simulink model "ArchModel"  (R2022a)
settings: Solver=VariableStepAuto  StartTime=0.0  StopTime=10.0  RelTol=1e-3
undefined symbols (not defined in the file or in its folder): Neg, Pos
undefined symbols (not defined in the file): DCL, EIS
settings Model: DataDictionary=DesignDictionary.sldd  Creator=mateu  LastModifiedBy=mateu

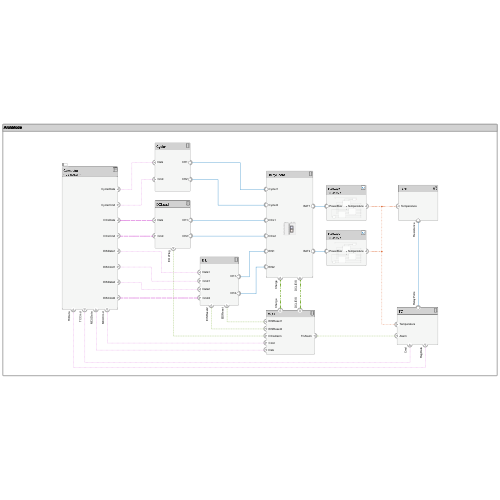
[thumbnail: Simulink's stored preview of the top-level diagram]
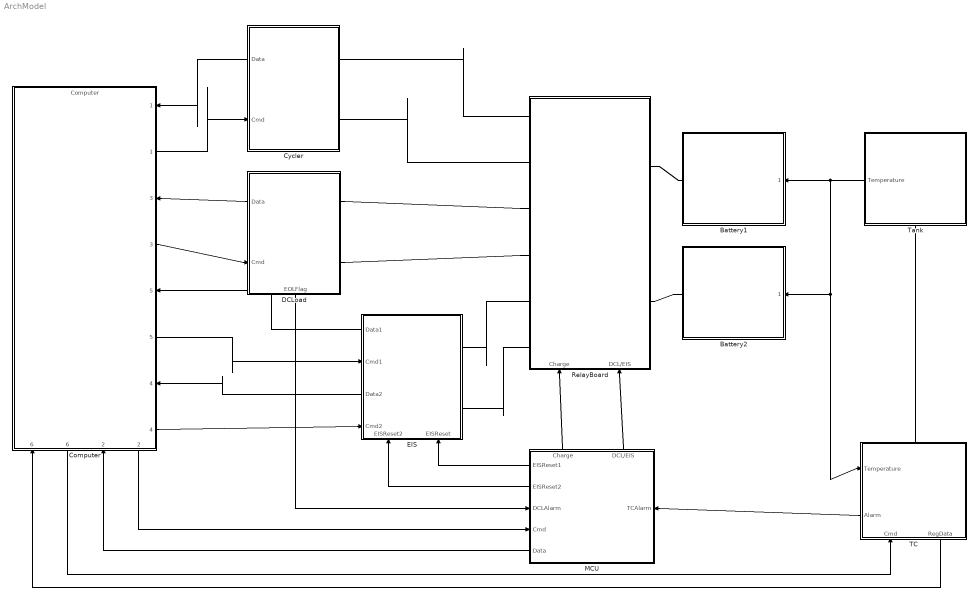
== system ArchModel ==
  Battery1 : Subsystem  ReferencedSubsystem=Battery
      settings: PortSchema="{\"entries\":[{\"content\":{\"headerSize\":26,\"margin\":15,\"minimumSpacing\":25,\"sides\":[{\"content\":{\"connectorIds\":[\"LConn1\"]},\"type\":\"ConnectorPlacement.EquallySpacedRectSide\",\"uuid\":\"7293e18d-b59a-4d1c-a013-b44ef7d38755\"},{\"content\":{\"connectorIds\":[\"In1\"],\"side\":\"RIGHT\"},\"type\":\"ConnectorPlacement.EquallySpacedRectSide\",\"uuid\":\"db41c958-7f9e-4f99-af5d-e3693d871bc2\"},{\"content\":{\"connectorIds\":[],\"side\":\"TOP\"},\"type\":\"ConnectorPlacement.EquallySpacedRectSide\",\"uuid\":\"914cc5b9-3cb5-4f98-b1a2-289c6929f7e4\"}]},\"type\":\"ConnectorPlacement.EquallySpacedConnector\",\"uuid\":\"372b3388-b57b-4345-a443-2207ebd52313\"}],\"packageUris\":[\"http://schema.mathworks.com/mf0/Connector/R2020b\"],\"version\":\"1.0\"}"
  Battery2 : Subsystem  ReferencedSubsystem=Battery
      settings: PortSchema="{\"entries\":[{\"content\":{\"headerSize\":26,\"margin\":15,\"minimumSpacing\":25,\"sides\":[{\"content\":{\"connectorIds\":[\"LConn1\"]},\"type\":\"ConnectorPlacement.EquallySpacedRectSide\",\"uuid\":\"7293e18d-b59a-4d1c-a013-b44ef7d38755\"},{\"content\":{\"connectorIds\":[\"In1\"],\"side\":\"RIGHT\"},\"type\":\"ConnectorPlacement.EquallySpacedRectSide\",\"uuid\":\"db41c958-7f9e-4f99-af5d-e3693d871bc2\"},{\"content\":{\"connectorIds\":[],\"side\":\"TOP\"},\"type\":\"ConnectorPlacement.EquallySpacedRectSide\",\"uuid\":\"914cc5b9-3cb5-4f98-b1a2-289c6929f7e4\"}]},\"type\":\"ConnectorPlacement.EquallySpacedConnector\",\"uuid\":\"372b3388-b57b-4345-a443-2207ebd52313\"}],\"packageUris\":[\"http://schema.mathworks.com/mf0/Connector/R2020b\"],\"version\":\"1.0\"}"
  Computer : ModelReference  ModelNameDialog=Computer  SimulationMode=Normal  ScheduleRates=on  ScheduleRatesWith=Schedule Editor  ModelReferenceVersion=1.3
      settings: PortSchema="{\"entries\":[{\"content\":{\"headerSize\":38,\"margin\":15,\"minimumSpacing\":25,\"sides\":[{\"content\":{\"connectorIds\":[]},\"type\":\"ConnectorPlacement.EquallySpacedRectSide\",\"uuid\":\"7293e18d-b59a-4d1c-a013-b44ef7d38755\"},{\"content\":{\"connectorIds\":[\"In1\",\"Out1\",\"In3\",\"Out3\",\"In5\",\"Out5\",\"In4\",\"Out4\"],\"side\":\"RIGHT\"},\"type\":\"ConnectorPlacement.EquallySpacedRectSide\",\"uuid\":\"db41c958-7f9e-4f99-af5d-e3693d871bc2\"},{\"content\":{\"connectorIds\":[],\"side\":\"TOP\"},\"type\":\"ConnectorPlacement.EquallySpacedRectSide\",\"uuid\":\"914cc5b9-3cb5-4f98-b1a2-289c6929f7e4\"},{\"content\":{\"connectorIds\":[\"In6\",\"Out6\",\"In2\",\"Out2\"],\"side\":\"BOTTOM\"},\"type\":\"ConnectorPlacement.EquallySpacedRectSide\",\"uuid\":\"ba0d90bc-7736-41e6-82f3-c99b67a5d224\"}]},\"type\":\"ConnectorPlacement.EquallySpacedConnector\",\"uuid\":\"372b3388-b57b-4345-a443-2207ebd52313\"}],\"packageUris\":[\"http://schema.mathworks.com/mf0/Connector/R2020b\"],\"version\":\"1.0\"}"
  Cycler : Subsystem
      settings: PortSchema="{\"entries\":[{\"content\":{\"headerSize\":26,\"margin\":15,\"minimumSpacing\":25,\"sides\":[{\"content\":{\"connectorIds\":[\"Out1\",\"In1\"]},\"type\":\"ConnectorPlacement.EquallySpacedRectSide\",\"uuid\":\"7293e18d-b59a-4d1c-a013-b44ef7d38755\"},{\"content\":{\"connectorIds\":[\"RConn1\",\"RConn2\"],\"side\":\"RIGHT\"},\"type\":\"ConnectorPlacement.EquallySpacedRectSide\",\"uuid\":\"db41c958-7f9e-4f99-af5d-e3693d871bc2\"},{\"content\":{\"connectorIds\":[],\"side\":\"TOP\"},\"type\":\"ConnectorPlacement.EquallySpacedRectSide\",\"uuid\":\"914cc5b9-3cb5-4f98-b1a2-289c6929f7e4\"}]},\"type\":\"ConnectorPlacement.EquallySpacedConnector\",\"uuid\":\"372b3388-b57b-4345-a443-2207ebd52313\"}],\"packageUris\":[\"http://schema.mathworks.com/mf0/Connector/R2020b\"],\"version\":\"1.0\"}"
  DCLoad : Subsystem
      settings: PortSchema="{\"entries\":[{\"content\":{\"headerSize\":26,\"margin\":15,\"minimumSpacing\":25,\"sides\":[{\"content\":{\"connectorIds\":[\"Out2\",\"In1\"]},\"type\":\"ConnectorPlacement.EquallySpacedRectSide\",\"uuid\":\"7293e18d-b59a-4d1c-a013-b44ef7d38755\"},{\"content\":{\"connectorIds\":[\"RConn1\",\"RConn2\"],\"side\":\"RIGHT\"},\"type\":\"ConnectorPlacement.EquallySpacedRectSide\",\"uuid\":\"db41c958-7f9e-4f99-af5d-e3693d871bc2\"},{\"content\":{\"connectorIds\":[],\"side\":\"TOP\"},\"type\":\"ConnectorPlacement.EquallySpacedRectSide\",\"uuid\":\"914cc5b9-3cb5-4f98-b1a2-289c6929f7e4\"},{\"content\":{\"connectorIds\":[\"Out1\"],\"side\":\"BOTTOM\"},\"type\":\"ConnectorPlacement.EquallySpacedRectSide\",\"uuid\":\"1b886045-7e55-48a4-a5ee-d0c1d4827f52\"}]},\"type\":\"ConnectorPlacement.EquallySpacedConnector\",\"uuid\":\"372b3388-b57b-4345-a443-2207ebd52313\"}],\"packageUris\":[\"http://schema.mathworks.com/mf0/Connector/R2020b\"],\"version\":\"1.0\"}"
  EIS : Subsystem
      settings: PortSchema="{\"entries\":[{\"content\":{\"headerSize\":26,\"margin\":15,\"minimumSpacing\":25,\"sides\":[{\"content\":{\"connectorIds\":[\"Out1\",\"In4\",\"Out2\",\"In3\"]},\"type\":\"ConnectorPlacement.EquallySpacedRectSide\",\"uuid\":\"7293e18d-b59a-4d1c-a013-b44ef7d38755\"},{\"content\":{\"connectorIds\":[\"RConn1\",\"RConn2\"],\"side\":\"RIGHT\"},\"type\":\"ConnectorPlacement.EquallySpacedRectSide\",\"uuid\":\"db41c958-7f9e-4f99-af5d-e3693d871bc2\"},{\"content\":{\"connectorIds\":[],\"side\":\"TOP\"},\"type\":\"ConnectorPlacement.EquallySpacedRectSide\",\"uuid\":\"914cc5b9-3cb5-4f98-b1a2-289c6929f7e4\"},{\"content\":{\"connectorIds\":[\"In1\",\"In2\"],\"side\":\"BOTTOM\"},\"type\":\"ConnectorPlacement.EquallySpacedRectSide\",\"uuid\":\"72880b12-21e3-4cc6-8f88-1609d84de5b0\"}]},\"type\":\"ConnectorPlacement.EquallySpacedConnector\",\"uuid\":\"372b3388-b57b-4345-a443-2207ebd52313\"}],\"packageUris\":[\"http://schema.mathworks.com/mf0/Connector/R2020b\"],\"version\":\"1.0\"}"
  MCU : Subsystem
      settings: PortSchema="{\"entries\":[{\"content\":{\"headerSize\":26,\"margin\":15,\"minimumSpacing\":25,\"sides\":[{\"content\":{\"connectorIds\":[\"Out1\",\"Out2\",\"In1\",\"In2\",\"Out3\"]},\"type\":\"ConnectorPlacement.EquallySpacedRectSide\",\"uuid\":\"7293e18d-b59a-4d1c-a013-b44ef7d38755\"},{\"content\":{\"connectorIds\":[\"In3\"],\"side\":\"RIGHT\"},\"type\":\"ConnectorPlacement.EquallySpacedRectSide\",\"uuid\":\"db41c958-7f9e-4f99-af5d-e3693d871bc2\"},{\"content\":{\"connectorIds\":[\"Out4\",\"Out5\"],\"side\":\"TOP\"},\"type\":\"ConnectorPlacement.EquallySpacedRectSide\",\"uuid\":\"914cc5b9-3cb5-4f98-b1a2-289c6929f7e4\"},{\"content\":{\"connectorIds\":[],\"side\":\"BOTTOM\"},\"type\":\"ConnectorPlacement.EquallySpacedRectSide\",\"uuid\":\"f4beb314-4f1a-4ac8-9406-4b22f31c5233\"}]},\"type\":\"ConnectorPlacement.EquallySpacedConnector\",\"uuid\":\"372b3388-b57b-4345-a443-2207ebd52313\"}],\"packageUris\":[\"http://schema.mathworks.com/mf0/Connector/R2020b\"],\"version\":\"1.0\"}"
  RelayBoard : Subsystem
      settings: PortSchema="{\"entries\":[{\"content\":{\"headerSize\":26,\"margin\":15,\"minimumSpacing\":25,\"sides\":[{\"content\":{\"connectorIds\":[\"LConn1\",\"LConn2\",\"LConn3\",\"LConn4\",\"LConn5\",\"LConn6\"]},\"type\":\"ConnectorPlacement.EquallySpacedRectSide\",\"uuid\":\"7293e18d-b59a-4d1c-a013-b44ef7d38755\"},{\"content\":{\"connectorIds\":[\"RConn1\",\"RConn2\"],\"side\":\"RIGHT\"},\"type\":\"ConnectorPlacement.EquallySpacedRectSide\",\"uuid\":\"db41c958-7f9e-4f99-af5d-e3693d871bc2\"},{\"content\":{\"connectorIds\":[],\"side\":\"TOP\"},\"type\":\"ConnectorPlacement.EquallySpacedRectSide\",\"uuid\":\"914cc5b9-3cb5-4f98-b1a2-289c6929f7e4\"},{\"content\":{\"connectorIds\":[\"In1\",\"In2\"],\"side\":\"BOTTOM\"},\"type\":\"ConnectorPlacement.EquallySpacedRectSide\",\"uuid\":\"a2b6a4b5-2cdb-4351-85fd-bf0b4fbbff2a\"}]},\"type\":\"ConnectorPlacement.EquallySpacedConnector\",\"uuid\":\"372b3388-b57b-4345-a443-2207ebd52313\"}],\"packageUris\":[\"http://schema.mathworks.com/mf0/Connector/R2020b\"],\"version\":\"1.0\"}"
  TC : Subsystem
      settings: PortSchema="{\"entries\":[{\"content\":{\"headerSize\":26,\"margin\":15,\"minimumSpacing\":25,\"sides\":[{\"content\":{\"connectorIds\":[\"In1\",\"Out1\"]},\"type\":\"ConnectorPlacement.EquallySpacedRectSide\",\"uuid\":\"7293e18d-b59a-4d1c-a013-b44ef7d38755\"},{\"content\":{\"connectorIds\":[],\"side\":\"RIGHT\"},\"type\":\"ConnectorPlacement.EquallySpacedRectSide\",\"uuid\":\"db41c958-7f9e-4f99-af5d-e3693d871bc2\"},{\"content\":{\"connectorIds\":[\"RConn1\"],\"side\":\"TOP\"},\"type\":\"ConnectorPlacement.EquallySpacedRectSide\",\"uuid\":\"914cc5b9-3cb5-4f98-b1a2-289c6929f7e4\"},{\"content\":{\"connectorIds\":[\"In2\",\"Out2\"],\"side\":\"BOTTOM\"},\"type\":\"ConnectorPlacement.EquallySpacedRectSide\",\"uuid\":\"030fdba4-d38a-4bc7-aed2-f5c752c86f7c\"}]},\"type\":\"ConnectorPlacement.EquallySpacedConnector\",\"uuid\":\"372b3388-b57b-4345-a443-2207ebd52313\"}],\"packageUris\":[\"http://schema.mathworks.com/mf0/Connector/R2020b\"],\"version\":\"1.0\"}"
  Tank : Subsystem
      settings: PortSchema="{\"entries\":[{\"content\":{\"headerSize\":26,\"margin\":15,\"minimumSpacing\":25,\"sides\":[{\"content\":{\"connectorIds\":[\"Out1\"]},\"type\":\"ConnectorPlacement.EquallySpacedRectSide\",\"uuid\":\"7293e18d-b59a-4d1c-a013-b44ef7d38755\"},{\"content\":{\"connectorIds\":[],\"side\":\"RIGHT\"},\"type\":\"ConnectorPlacement.EquallySpacedRectSide\",\"uuid\":\"db41c958-7f9e-4f99-af5d-e3693d871bc2\"},{\"content\":{\"connectorIds\":[],\"side\":\"TOP\"},\"type\":\"ConnectorPlacement.EquallySpacedRectSide\",\"uuid\":\"914cc5b9-3cb5-4f98-b1a2-289c6929f7e4\"},{\"content\":{\"connectorIds\":[\"LConn1\"],\"side\":\"BOTTOM\"},\"type\":\"ConnectorPlacement.EquallySpacedRectSide\",\"uuid\":\"2d7b9bd5-98de-4a16-aa91-7572a08146ef\"}]},\"type\":\"ConnectorPlacement.EquallySpacedConnector\",\"uuid\":\"372b3388-b57b-4345-a443-2207ebd52313\"}],\"packageUris\":[\"http://schema.mathworks.com/mf0/Connector/R2020b\"],\"version\":\"1.0\"}"
  wires:
  Tank/1(Temperature) -> TC/1(Temperature), Battery2/1, Battery1/1
  MCU/4(Charge) -> RelayBoard/1(Charge)
  MCU/5(DCL/EIS) -> RelayBoard/2(DCL/EIS)
  TC/1(Alarm) -> MCU/3(TCAlarm)
  MCU/1(EISReset1) -> EIS/2(EISReset)
  DCLoad/1(EOLFlag) -> MCU/1(DCLAlarm)
  MCU/2(EISReset2) -> EIS/1(EISReset2)
  Cycler/1(Data) -> Computer/1
  DCLoad/2(Data) -> Computer/3
  EIS/1(Data1) -> Computer/5
  EIS/2(Data2) -> Computer/4
  MCU/3(Data) -> Computer/2
  TC/2(RegData) -> Computer/6
  Computer/1 -> Cycler/1(Cmd)
  Computer/3 -> DCLoad/1(Cmd)
  Computer/5 -> EIS/4(Cmd1)
  Computer/4 -> EIS/3(Cmd2)
  Computer/2 -> MCU/2(Cmd)
  Computer/6 -> TC/2(Cmd)
  connections:
  RelayBoard/RConn1 -- Battery1/LConn1
  Battery2/LConn1 -- RelayBoard/RConn2
  TC/RConn1 -- Tank/LConn1
  RelayBoard/LConn3 -- DCLoad/RConn1
  RelayBoard/LConn4 -- DCLoad/RConn2
  RelayBoard/LConn5 -- EIS/RConn1
  RelayBoard/LConn6 -- EIS/RConn2
  RelayBoard/LConn1 -- Cycler/RConn1
  RelayBoard/LConn2 -- Cycler/RConn2

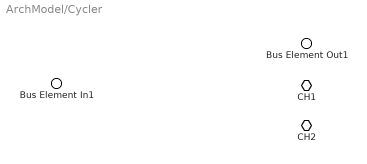
== system ArchModel/Cycler ==
  Bus Element In1 : Inport  PortName=Cmd
  CH1 : PMIOPort  Side=Right  ConnectionType=Bus: DCBus
  CH2 : PMIOPort  Port=2  Side=Right  ConnectionType=Bus: DCBus
  Bus Element Out1 : Outport  PortName=Data

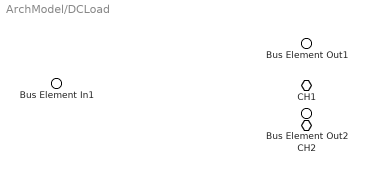
== system ArchModel/DCLoad ==
  Bus Element In1 : Inport  PortName=Cmd
  CH1 : PMIOPort  Side=Right  ConnectionType=Bus: DCBus
  CH2 : PMIOPort  Port=2  Side=Right  ConnectionType=Bus: DCBus
  Bus Element Out1 : Outport  PortName=EOLFlag
  Bus Element Out2 : Outport  Port=2  PortName=Data

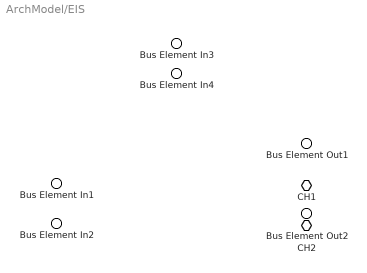
== system ArchModel/EIS ==
  Bus Element In4 : Inport  PortName=EISReset2
  Bus Element In1 : Inport  Port=2  PortName=EISReset
  Bus Element In3 : Inport  Port=3  PortName=Cmd2
  Bus Element In2 : Inport  Port=4  PortName=Cmd1
  CH1 : PMIOPort  Side=Right  ConnectionType=Bus: DCBus
  CH2 : PMIOPort  Port=2  Side=Right  ConnectionType=Bus: DCBus
  Bus Element Out1 : Outport  PortName=Data1
  Bus Element Out2 : Outport  Port=2  PortName=Data2

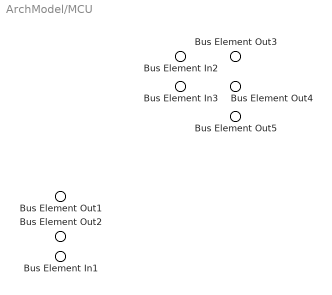
== system ArchModel/MCU ==
  Bus Element In2 : Inport  PortName=DCLAlarm
  Bus Element In3 : Inport  Port=2  PortName=Cmd
  Bus Element In1 : Inport  Port=3  PortName=TCAlarm
  Bus Element Out3 : Outport  PortName=EISReset1
  Bus Element Out5 : Outport  Port=2  PortName=EISReset2
  Bus Element Out4 : Outport  Port=3  PortName=Data
  Bus Element Out1 : Outport  Port=4  PortName=Charge
  Bus Element Out2 : Outport  Port=5  PortName=DCL/EIS

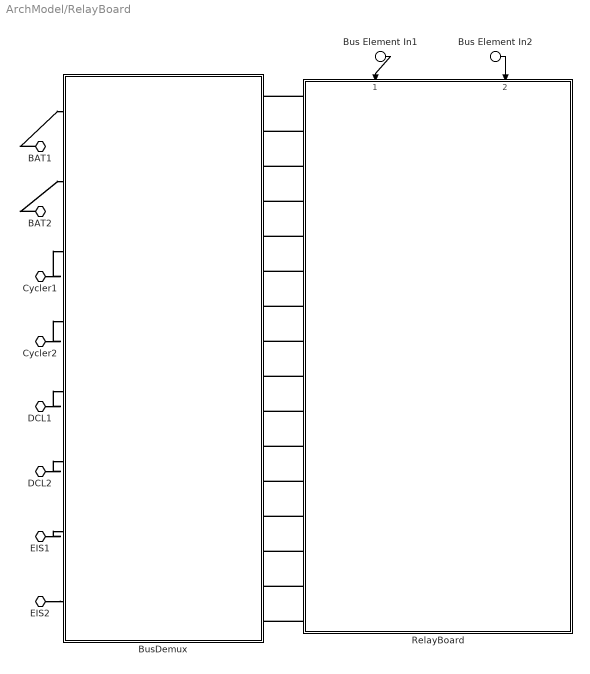
== system ArchModel/RelayBoard ==
  Bus Element In1 : Inport  PortName=Charge
  Bus Element In2 : Inport  Port=2  PortName=DCL/EIS
  BusDemux : Subsystem
      settings: PortSchema="{\"entries\":[{\"content\":{\"headerSize\":26,\"margin\":15,\"minimumSpacing\":25,\"sides\":[{\"content\":{\"connectorIds\":[\"LConn1\",\"LConn2\",\"LConn3\",\"LConn4\",\"LConn5\",\"LConn6\",\"LConn7\",\"LConn8\"]},\"type\":\"ConnectorPlacement.EquallySpacedRectSide\",\"uuid\":\"7293e18d-b59a-4d1c-a013-b44ef7d38755\"},{\"content\":{\"connectorIds\":[\"RConn3\",\"RConn4\",\"RConn5\",\"RConn6\",\"RConn7\",\"RConn2\",\"RConn8\",\"RConn9\",\"RConn10\",\"RConn11\",\"RConn12\",\"RConn13\",\"RConn14\",\"RConn1\",\"RConn15\",\"RConn16\"],\"side\":\"RIGHT\"},\"type\":\"ConnectorPlacement.EquallySpacedRectSide\",\"uuid\":\"db41c958-7f9e-4f99-af5d-e3693d871bc2\"},{\"content\":{\"connectorIds\":[],\"side\":\"TOP\"},\"type\":\"ConnectorPlacement.EquallySpacedRectSide\",\"uuid\":\"914cc5b9-3cb5-4f98-b1a2-289c6929f7e4\"},{\"content\":{\"connectorIds\":[],\"side\":\"BOTTOM\"},\"type\":\"ConnectorPlacement.EquallySpacedRectSide\",\"uuid\":\"78d1bca9-ec29-4602-b948-27979d0c9b82\"}]},\"type\":\"ConnectorPlacement.EquallySpacedConnector\",\"uuid\":\"372b3388-b57b-4345-a443-2207ebd52313\"}],\"packageUris\":[\"http://schema.mathworks.com/mf0/Connector/R2020b\"],\"version\":\"1.0\"}"
  RelayBoard : Subsystem  ReferencedSubsystem=RelayBoard
      settings: PortSchema="{\"entries\":[{\"content\":{\"headerSize\":26,\"margin\":15,\"minimumSpacing\":25,\"sides\":[{\"content\":{\"connectorIds\":[\"LConn1\",\"LConn2\",\"LConn3\",\"LConn4\",\"LConn5\",\"LConn6\",\"LConn7\",\"LConn8\",\"RConn1\",\"RConn2\",\"RConn3\",\"RConn4\",\"RConn5\",\"RConn6\",\"RConn7\",\"RConn8\"]},\"type\":\"ConnectorPlacement.EquallySpacedRectSide\",\"uuid\":\"7293e18d-b59a-4d1c-a013-b44ef7d38755\"},{\"content\":{\"connectorIds\":[],\"side\":\"RIGHT\"},\"type\":\"ConnectorPlacement.EquallySpacedRectSide\",\"uuid\":\"db41c958-7f9e-4f99-af5d-e3693d871bc2\"},{\"content\":{\"connectorIds\":[\"In1\",\"In2\"],\"side\":\"TOP\"},\"type\":\"ConnectorPlacement.EquallySpacedRectSide\",\"uuid\":\"914cc5b9-3cb5-4f98-b1a2-289c6929f7e4\"}]},\"type\":\"ConnectorPlacement.EquallySpacedConnector\",\"uuid\":\"372b3388-b57b-4345-a443-2207ebd52313\"}],\"packageUris\":[\"http://schema.mathworks.com/mf0/Connector/R2020b\"],\"version\":\"1.0\"}"
  BAT1 : PMIOPort  Side=Right  ConnectionType=Bus: DCBus
  BAT2 : PMIOPort  Port=2  Side=Right  ConnectionType=Bus: DCBus
  Cycler1 : PMIOPort  Port=3  Side=Left  ConnectionType=Bus: DCBus
  Cycler2 : PMIOPort  Port=4  Side=Left  ConnectionType=Bus: DCBus
  DCL1 : PMIOPort  Port=5  Side=Left  ConnectionType=Bus: DCBus
  DCL2 : PMIOPort  Port=6  Side=Left  ConnectionType=Bus: DCBus
  EIS1 : PMIOPort  Port=7  Side=Left  ConnectionType=Bus: DCBus
  EIS2 : PMIOPort  Port=8  Side=Left  ConnectionType=Bus: DCBus
  wires:
  Bus Element In1/1 -> RelayBoard/1
  Bus Element In2/1 -> RelayBoard/2
  connections:
  BAT1/RConn1 -- BusDemux/LConn1
  BAT2/RConn1 -- BusDemux/LConn2
  Cycler1/RConn1 -- BusDemux/LConn3
  Cycler2/RConn1 -- BusDemux/LConn4
  DCL1/RConn1 -- BusDemux/LConn5
  DCL2/RConn1 -- BusDemux/LConn6
  EIS1/RConn1 -- BusDemux/LConn7
  EIS2/RConn1 -- BusDemux/LConn8
  RelayBoard/LConn1 -- BusDemux/RConn3
  RelayBoard/LConn2 -- BusDemux/RConn4
  RelayBoard/LConn3 -- BusDemux/RConn5
  RelayBoard/LConn4 -- BusDemux/RConn6
  RelayBoard/LConn5 -- BusDemux/RConn7
  RelayBoard/LConn6 -- BusDemux/RConn2
  RelayBoard/LConn7 -- BusDemux/RConn8
  RelayBoard/LConn8 -- BusDemux/RConn9
  RelayBoard/RConn1 -- BusDemux/RConn10
  RelayBoard/RConn2 -- BusDemux/RConn11
  RelayBoard/RConn3 -- BusDemux/RConn12
  RelayBoard/RConn4 -- BusDemux/RConn13
  RelayBoard/RConn5 -- BusDemux/RConn14
  RelayBoard/RConn6 -- BusDemux/RConn1
  RelayBoard/RConn7 -- BusDemux/RConn15
  RelayBoard/RConn8 -- BusDemux/RConn16

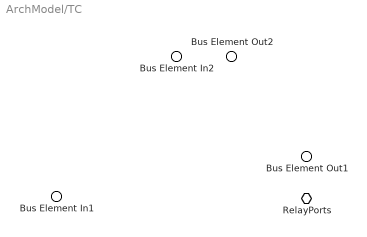
== system ArchModel/TC ==
  Bus Element In2 : Inport  PortName=Temperature
  Bus Element In1 : Inport  Port=2  PortName=Cmd
  RelayPorts : PMIOPort  Side=Right  ConnectionType=Bus: ACBus
  Bus Element Out2 : Outport  PortName=Alarm
  Bus Element Out1 : Outport  Port=2  PortName=RegData

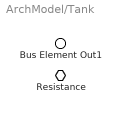
== system ArchModel/Tank ==
  Resistance : PMIOPort  Side=Left  ConnectionType=Bus: ACBus
  Bus Element Out1 : Outport  PortName=Temperature

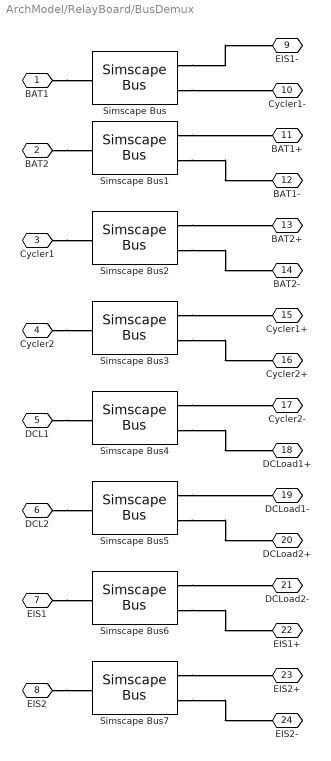
== system ArchModel/RelayBoard/BusDemux ==
  Simscape Bus{,1..7} (8 alike) : SimscapeBus  HierarchyStrings=Pos;Neg  ConnectionType=Bus: DCBus
  BAT1 : PMIOPort  Side=Left  ConnectionType=Bus: DCBus
  BAT2 : PMIOPort  Port=2  Side=Left  ConnectionType=Bus: DCBus
  Cycler1 : PMIOPort  Port=3  Side=Left  ConnectionType=Bus: DCBus
  Cycler2 : PMIOPort  Port=4  Side=Left  ConnectionType=Bus: DCBus
  DCL1 : PMIOPort  Port=5  Side=Left  ConnectionType=Bus: DCBus
  DCL2 : PMIOPort  Port=6  Side=Left  ConnectionType=Bus: DCBus
  EIS1 : PMIOPort  Port=7  Side=Left  ConnectionType=Bus: DCBus
  EIS2 : PMIOPort  Port=8  Side=Left  ConnectionType=Bus: DCBus
  EIS1- : PMIOPort  Port=9  Side=Right
  Cycler1- : PMIOPort  Port=10  Side=Right
  BAT1+ : PMIOPort  Port=11  Side=Right
  BAT1- : PMIOPort  Port=12  Side=Right
  BAT2+ : PMIOPort  Port=13  Side=Right
  BAT2- : PMIOPort  Port=14  Side=Right
  Cycler1+ : PMIOPort  Port=15  Side=Right
  Cycler2+ : PMIOPort  Port=16  Side=Right
  Cycler2- : PMIOPort  Port=17  Side=Right
  DCLoad1+ : PMIOPort  Port=18  Side=Right
  DCLoad1- : PMIOPort  Port=19  Side=Right
  DCLoad2+ : PMIOPort  Port=20  Side=Right
  DCLoad2- : PMIOPort  Port=21  Side=Right
  EIS1+ : PMIOPort  Port=22  Side=Right
  EIS2+ : PMIOPort  Port=23  Side=Right
  EIS2- : PMIOPort  Port=24  Side=Right
  connections:
  BAT1/RConn1 -- Simscape Bus/RConn1
  Simscape Bus/LConn1 -- EIS1-/RConn1
  Simscape Bus/LConn2 -- Cycler1-/RConn1
  BAT2/RConn1 -- Simscape Bus1/RConn1
  Simscape Bus1/LConn1 -- BAT1+/RConn1
  Simscape Bus1/LConn2 -- BAT1-/RConn1
  Simscape Bus2/LConn1 -- BAT2+/RConn1
  Simscape Bus2/LConn2 -- BAT2-/RConn1
  Simscape Bus3/LConn1 -- Cycler1+/RConn1
  Simscape Bus3/LConn2 -- Cycler2+/RConn1
  Simscape Bus4/LConn1 -- Cycler2-/RConn1
  Simscape Bus4/LConn2 -- DCLoad1+/RConn1
  Simscape Bus5/LConn1 -- DCLoad1-/RConn1
  Simscape Bus5/LConn2 -- DCLoad2+/RConn1
  Simscape Bus6/LConn1 -- DCLoad2-/RConn1
  Simscape Bus6/LConn2 -- EIS1+/RConn1
  Simscape Bus7/LConn1 -- EIS2+/RConn1
  Simscape Bus7/LConn2 -- EIS2-/RConn1
  Cycler1/RConn1 -- Simscape Bus2/RConn1
  Cycler2/RConn1 -- Simscape Bus3/RConn1
  DCL1/RConn1 -- Simscape Bus4/RConn1
  DCL2/RConn1 -- Simscape Bus5/RConn1
  EIS1/RConn1 -- Simscape Bus6/RConn1
  EIS2/RConn1 -- Simscape Bus7/RConn1
